simulink model "tempo"  (R2012b)
settings: Solver=ode45  StartTime=0.0  StopTime=20  RelTol=1e-3
libraries: fuzblock x1
settings Model: Creator=2Filipek  LastModifiedBy=Amadeusz

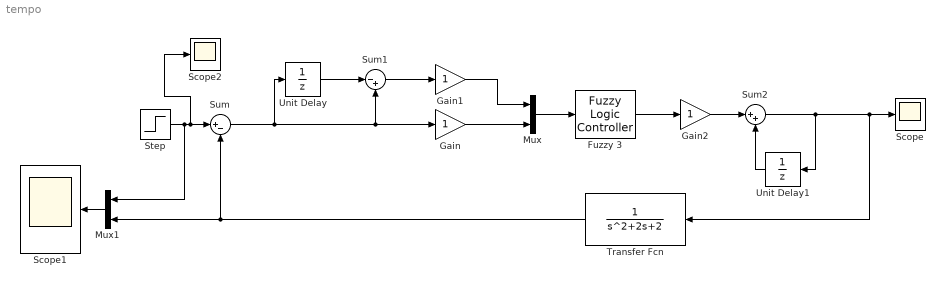
== system tempo ==
  Fuzzy 3 : fuzblock/Fuzzy Logic  Controller  fis=['fuzzy_3']
  Gain : Gain
  Gain1 : Gain
  Gain2 : Gain
  Mux : Mux  Inputs=2
  Mux1 : Mux  Inputs=2
  Scope : Scope
  Scope1 : Scope
      settings: TimeRange=2  YMin=-0.5030181086519105  YMax=0.3420523138833005
  Scope2 : Scope
      settings: SaveName=ScopeData2
  Step : Step  SampleTime=0
  Sum : Sum  Inputs=|+-
  Sum1 : Sum  Inputs=|-+
  Sum2 : Sum  Inputs=|++
  Transfer Fcn : TransferFcn  Denominator=[1 2 2]
  Unit Delay : UnitDelay
  Unit Delay1 : UnitDelay
  wires:
  Mux/1 -> Fuzzy 3/1
  Sum/1 -> Unit Delay/1, Sum1/2, Gain/1
  Unit Delay/1 -> Sum1/1
  Gain/1 -> Mux/2
  Sum1/1 -> Gain1/1
  Gain1/1 -> Mux/1
  Fuzzy 3/1 -> Gain2/1
  Gain2/1 -> Sum2/1
  Unit Delay1/1 -> Sum2/2
  Sum2/1 -> Unit Delay1/1, Scope/1, Transfer Fcn/1
  Transfer Fcn/1 -> Mux1/2, Sum/2
  Step/1 -> Mux1/1, Scope2/1, Sum/1
  Mux1/1 -> Scope1/1
